simulink model "examen"  (R2017a)
settings: Solver=VariableStepAuto  StartTime=0.0  StopTime=10.0  RelTol=1e-3
settings Model: Creator=firass2019  LastModifiedBy=firass2019

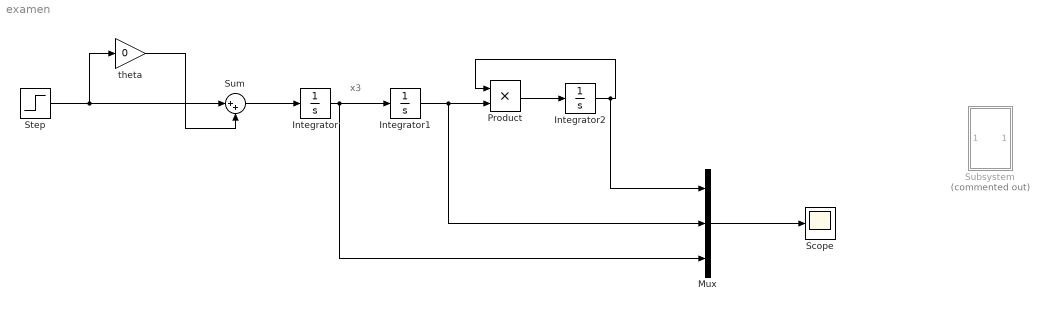
== system examen ==
  note: x3
  Integrator : Integrator
  Integrator1 : Integrator  InitialCondition=1
  Integrator2 : Integrator
  Mux : Mux  Inputs=3
  Product : Product
  Scope : Scope
  Step : Step  Time=0  SampleTime=0
  Subsystem : Subsystem  Commented=on
  Sum : Sum  Inputs=|++
  "theta " : Gain  Gain=0
  wires:
  Sum/1 -> Integrator/1
  Step/1 -> "theta "/1, Sum/1
  "theta "/1 -> Sum/2
  Integrator/1 -> Mux/3, Integrator1/1
  Integrator1/1 -> Mux/2, Product/2
  Product/1 -> Integrator2/1
  Integrator2/1 -> Mux/1, Product/1
  Mux/1 -> Scope/1

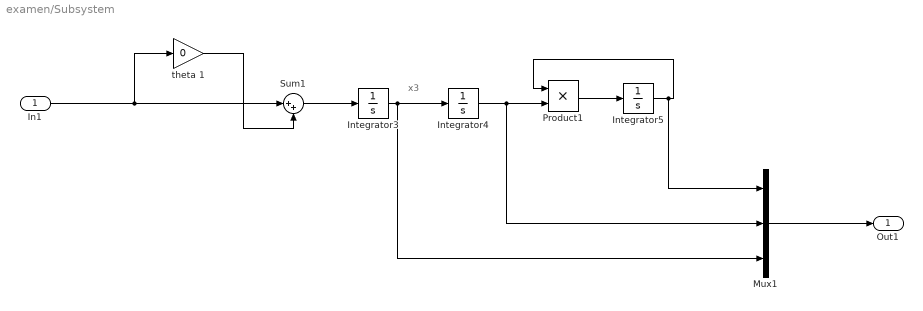
== system examen/Subsystem ==
  note: x3
  In1 : Inport
  Integrator3 : Integrator
  Integrator4 : Integrator
  Integrator5 : Integrator
  Mux1 : Mux  Inputs=3
  Product1 : Product
  Sum1 : Sum  Inputs=|++
  theta 1 : Gain  Gain=0
  Out1 : Outport
  wires:
  Integrator3/1 -> Mux1/3, Integrator4/1
  In1/1 -> theta 1/1, Sum1/1
  theta 1/1 -> Sum1/2
  Integrator4/1 -> Mux1/2, Product1/2
  Sum1/1 -> Integrator3/1
  Integrator5/1 -> Mux1/1, Product1/1
  Mux1/1 -> Out1/1
  Product1/1 -> Integrator5/1
